simulink model "Demo_DSRC_BSM_I_and_II_Message_cs"  (Simulink 7.6)
settings: Solver=ode5  SolverMode=SingleTasking  StartTime=0.0  StopTime=40  FixedStep=1/20  RelTol=1e-3
PreLoadFcn:
  | check_NUTS_defined;
  | 
  | assignin('base',['model_closed_' bdroot],false);
InitFcn:
  | PreScanExperimentInitFcn(bdroot)
StopFcn:
  | PreScanExperimentStopFcn(bdroot)
libraries: simulink x9, PreScanSimulinkLibrary x8, PreScanUsefulBlocks x5, simulink_extras x1
(part 2 of 3)

== system Demo_DSRC_BSM_I_and_II_Message_cs/Mazda_RX8_1/Basic Safety Message II ==
  ThrottlePosition : Inport
  ExteriorLights : Inport  Port=2
  CrumbData : Inport  Port=3
  itemCnt : Inport  Port=4
  Confidence : Inport  Port=5
  RadiusOfCurve : Inport  Port=6
  EventFlag : Inport  Port=7
  BSM-II Creator : Subsystem  InitFcn=|  StopFcn=|
      InitFcn=|
      | clear elems;
      | elems(1) = Simulink.BusElement;
      | elems(1).Name = 'VehicleStatus';
      | elems(1).Dimensions = 1;
      | elems(1).DataType = 'VehicleStatus';
      | elems(1).SampleTime = -1;
      | elems(1).Complexity = 'real';
      | elems(1).SamplingMode = 'Sample based';
      | elems(2) = Simulink.BusElement;
      | elems(2).Name = 'VehicleSafetyExtension';
      | elems(2).Dimensions = 1;
      | elems(2).DataType = 'VehicleSafetyExtension';
      | elems(2).SampleTime = -1;
      | elems(2).Complexity = 'real';
      | elems(2).SamplingMode = 'Sample based';
      | BSMII = Simulink.Bus;
      | BSMII.HeaderFile = '';
      | BSMII.Description = sprintf('BSMII message set');
      | BSMII.Elements = elems;
      | assignin('base', 'BSMII', BSMII)
      | % Bus object: PathHistory
      | clear elems;
      | elems(1) = Simulink.BusElement;
      | elems(1).Name = 'CrumbData';
      | elems(1).Dimensions = 184;
      | elems(1).DataType = 'uint8';
      | elems(1).SampleTime = -1;
      | elems(1).Complexity = 'real';
      | elems(1).SamplingMode = 'Sample based';
      | elems(2) = Simulink.BusElement;
      | elems(2).Name = 'itemCnt';
      | elems(2).Dimensions = 1;
      | elems(2).DataType = 'uint8';
      | elems(2).SampleTime = -1;
      | elems(2).Complexity = 'real';
      | elems(2).SamplingMode = 'Sample based';
      | PathHistory = Simulink.Bus;
      | PathHistory.HeaderFile = '';
      | PathHistory.Description = sprintf('');
      | PathHistory.Elements = elems;
      | assignin('base', 'PathHistory', PathHistory)
      | % Bus object: PathPrediction
      | clear elems;
      | elems(1) = Simulink.BusElement;
      | elems(1).Name = 'Confidence';
      | elems(1).Dimensions = 1;
      | elems(1).DataType = 'uint8';
      | elems(1).SampleTime = -1;
      | elems(1).Complexity = 'real';
      | elems(1).SamplingMode = 'Sample based';
      | elems(2) = Simulink.BusElement;
      | elems(2).Name = 'RadiusOfCurve';
      | elems(2).Dimensions = 1;
      | elems(2).DataType = 'int16';
      | elems(2).SampleTime = -1;
      | elems(2).Complexity = 'real';
      | elems(2).SamplingMode = 'Sample based';
      | PathPrediction = Simulink.Bus;
      | PathPrediction.HeaderFile = '';
      | PathPrediction.Description = sprintf('');
      | PathPrediction.Elements = elems;
      | assignin('base', 'PathPrediction', PathPrediction)
      | % Bus object: VehicleSafetyExtension
      | clear elems;
      | elems(1) = Simulink.BusElement;
      | elems(1).Name = 'PathPrediction';
      | elems(1).Dimensions = 1;
      | elems(1).DataType = 'PathPrediction';
      | elems(1).SampleTime = -1;
      | elems(1).Complexity = 'real';
      | elems(1).SamplingMode = 'Sample based';
      | elems(2) = Simulink.BusElement;
      | elems(2).Name = 'PathHistory';
      | elems(2).Dimensions = 1;
      | elems(2).DataType = 'PathHistory';
      | elems(2).SampleTime = -1;
      | elems(2).Complexity = 'real';
      | elems(2).SamplingMode = 'Sample based';
      | elems(3) = Simulink.BusElement;
      | elems(3).Name = 'EventFlag';
      | elems(3).Dimensions = 1;
      | elems(3).DataType = 'uint32';
      | elems(3).SampleTime = -1;
      | elems(3).Complexity = 'real';
      | elems(3).SamplingMode = 'Sample based';
      | VehicleSafetyExtension = Simulink.Bus;
      | VehicleSafetyExtension.HeaderFile = '';
      | VehicleSafetyExtension.Description = sprintf('');
      | VehicleSafetyExtension.Elements = elems;
      | assignin('base', 'VehicleSafetyExtension', VehicleSafetyExtension)
      | % Bus object: VehicleStatus
      | clear elems;
      | elems(1) = Simulink.BusElement;
      | elems(1).Name = 'ThrottlePosition';
      | elems(1).Dimensions = 1;
      | elems(1).DataType = 'uint8';
      | elems(1).SampleTime = -1;
      | elems(1).Complexity = 'real';
      | elems(1).SamplingMode = 'Sample based';
      | elems(2) = Simulink.BusElement;
      | elems(2).Name = 'ExteriorLights';
      | elems(2).Dimensions = 1;
      | elems(2).DataType = 'uint8';
      | elems(2).SampleTime = -1;
      | elems(2).Complexity = 'real';
      | elems(2).SamplingMode = 'Sample based';
      | VehicleStatus = Simulink.Bus;
      | VehicleStatus.HeaderFile = '';
      | VehicleStatus.Description = sprintf('');
      | VehicleStatus.Elements = elems;
      | assignin('base', 'VehicleStatus', VehicleStatus)
      StopFcn=|
      | clear BSMII
      | clear PathHistory
      | clear PathPrediction
      | clear VehicleSafetyExtension
      | clear VehicleStatus
      | clear elems
  BSM-II Unpacker : Subsystem
  Bus Creator : BusCreator  Inputs=8
  Enabled Basic Safety Message I and II : Subsystem
  BSMII : Outport
  wires:
  Enabled Basic Safety Message I and II/8(CrumbData out) -> Bus Creator/8  "CrumbData"
  Enabled Basic Safety Message I and II/7(Throttle position out) -> Bus Creator/7  "ThrottlePosition"
  Enabled Basic Safety Message I and II/6(Exterior lights out) -> Bus Creator/6  "ExteriorLights"
  Enabled Basic Safety Message I and II/5(Confidence out) -> Bus Creator/5  "Confidence"
  Enabled Basic Safety Message I and II/4(radius of Curve out) -> Bus Creator/4  "RadiusOfCurve"
  Enabled Basic Safety Message I and II/3(item Count out) -> Bus Creator/3  "itemCnt"
  Enabled Basic Safety Message I and II/2(Eventflag out) -> Bus Creator/2  "EventFlag"
  Enabled Basic Safety Message I and II/1(Enabled descriptor out) -> Bus Creator/1  "Enabled descriptor"
  BSM-II Creator/1(BSMII) -> BSM-II Unpacker/1(BSMII)
  Bus Creator/1 -> BSMII/1  "BSMII"
  ThrottlePosition/1 -> BSM-II Creator/1(ThrottlePositon)  "ThrottlePosition"
  ExteriorLights/1 -> BSM-II Creator/2(ExteriorLights)  "ExteriorLights"
  CrumbData/1 -> BSM-II Creator/3(CrumbData)  "CrumbData"
  itemCnt/1 -> BSM-II Creator/4(itemCnt)  "itemCnt"
  Confidence/1 -> BSM-II Creator/5(Confidence)  "Confidence"
  RadiusOfCurve/1 -> BSM-II Creator/6(RadiusOfCurve)  "RadiusOfCurve"
  EventFlag/1 -> BSM-II Creator/7(EventFlag)  "EventFlag"
  BSM-II Unpacker/1(Eventflag) -> Enabled Basic Safety Message I and II/1(Eventflag in)
  BSM-II Unpacker/2(itemCnt) -> Enabled Basic Safety Message I and II/2(itemCnt in)
  BSM-II Unpacker/3(RadiusOfCurve) -> Enabled Basic Safety Message I and II/3(radiusOfCurve in)
  BSM-II Unpacker/4(Confidence) -> Enabled Basic Safety Message I and II/4(Confidence in)
  BSM-II Unpacker/5(ExteriorLights) -> Enabled Basic Safety Message I and II/5(Exterior lights in)
  BSM-II Unpacker/6(ThrottlePosition) -> Enabled Basic Safety Message I and II/6(Throttle position in)
  BSM-II Unpacker/7(CrumbData_DoubleVector) -> Enabled Basic Safety Message I and II/7(CrumbData in)

== system Demo_DSRC_BSM_I_and_II_Message_cs/Mazda_RX8_1/DSRC Transmitter BSM I and II ==
  Data1 : Inport
  Enable : EnablePort  PropagateVarSize=During execution
  Always Enabled1 : Constant
  DSRC_T_BusAssignment : BusAssignment  Tag=BusDSRCT  AssignedSignals=spare_1,spare_2,spare_3,spare_4,spare_5,spare_6,spare_7,spare_8,spare_9,spare_10,spare_11,spare_12,spare_13,spare_14,spare_15,spare_16,spare_17,spare_18,spare_19,spare_20,spare_21,spare_22,spare_23,spare_24,spare_25,spare_26,spare_27,spare_28,spare_29,spare_30,spare_31,spare_32,spare_33,spare_34,spare_35,spare_36,spare_37,spare_38,spare_39,spare_40,spare_41,spare_42,spare_43,spare_44,spare_45,spare_46,spare_47,spare_48,spare_49,spare_50,spare_51,spare_52,spare_53,spare_54,spare_55,spare_56,spare_57,spare_58,spare_59,spare_60,spare_61,spare_62,spare_63
  DSRC_T_Mux : Subsystem  Tag=MuxDSRCT
      settings: DeleteFcn=PreScanBlockDeleteFcn;
      mask Type: PreScan Mux Block:
      mask Display:
      | port_label('input', 1, 'Warning signal ID')
      | port_label('input', 2, 'Maneuvre ID')
      | port_label('input', 3, 'Vehicle Type')
      | port_label('input', 4, 'Braking Capacity')
      | port_label('input', 5, 'Vehicle Size')
      | port_label('input', 6, 'spare')
  Demux : Demux  Outputs=63
  Ground_{4..8} (5 alike) : Ground
  DSRC_T : Outport  Tag=AntennaTOutport
  f() : Outport  Port=2  InitialOutput=[1]
  wires:
  DSRC_T_Mux/2(Out2) -> DSRC_T_BusAssignment/1  "L29"
  DSRC_T_Mux/1(Out1) -> DSRC_T/1  "l60"
  Ground_4/1 -> DSRC_T_Mux/1(warning_signal_id)  "l46"
  Ground_5/1 -> DSRC_T_Mux/2(maneuvre_id)  "l47"
  Ground_6/1 -> DSRC_T_Mux/3(vehicle_type)  "l48"
  Ground_7/1 -> DSRC_T_Mux/4(brakingcapacity)  "l49"
  Ground_8/1 -> DSRC_T_Mux/5(vehicle_size)  "l50"
  Demux/39 -> DSRC_T_BusAssignment/40
  Always Enabled1/1 -> f()/1
  DSRC_T_BusAssignment/1 -> DSRC_T_Mux/6(spare)  "l58"
  Demux/1 -> DSRC_T_BusAssignment/2  "MsgId"
  Demux/2 -> DSRC_T_BusAssignment/3  "MsgCount"
  Demux/3 -> DSRC_T_BusAssignment/4  "TempId"
  Demux/4 -> DSRC_T_BusAssignment/5  "SecMark"
  Demux/5 -> DSRC_T_BusAssignment/6  "Lateral"
  Demux/6 -> DSRC_T_BusAssignment/7  "Longitudinal"
  Demux/7 -> DSRC_T_BusAssignment/8  "Elevation"
  Demux/8 -> DSRC_T_BusAssignment/9  "Accuracy"
  Demux/9 -> DSRC_T_BusAssignment/10  "Transmission State"
  Demux/10 -> DSRC_T_BusAssignment/11  "Speed"
  Demux/11 -> DSRC_T_BusAssignment/12  "Heading"
  Demux/12 -> DSRC_T_BusAssignment/13  "Angle"
  Demux/13 -> DSRC_T_BusAssignment/14  "Longitudinal Acc"
  Demux/14 -> DSRC_T_BusAssignment/15  "Lateral Acc"
  Demux/15 -> DSRC_T_BusAssignment/16  "Veritical Acc"
  Demux/16 -> DSRC_T_BusAssignment/17  "Yaw rate"
  Demux/17 -> DSRC_T_BusAssignment/18  "Brakes"
  Demux/18 -> DSRC_T_BusAssignment/19  "Vehicle Width"
  Demux/19 -> DSRC_T_BusAssignment/20  "Vehicle Height"
  Demux/20 -> DSRC_T_BusAssignment/21  "Enabled_Descriptor"
  Demux/21 -> DSRC_T_BusAssignment/22  "Eventflag"
  Demux/22 -> DSRC_T_BusAssignment/23  "itemCnt"
  Demux/23 -> DSRC_T_BusAssignment/24  "radiusOfCurve"
  Demux/24 -> DSRC_T_BusAssignment/25  "confidence"
  Demux/25 -> DSRC_T_BusAssignment/26  "Exterior lights"
  Demux/26 -> DSRC_T_BusAssignment/27  "Throttle position"
  Demux/27 -> DSRC_T_BusAssignment/28
  Demux/28 -> DSRC_T_BusAssignment/29
  Demux/29 -> DSRC_T_BusAssignment/30
  Data1/1 -> Demux/1
  Demux/30 -> DSRC_T_BusAssignment/31
  Demux/31 -> DSRC_T_BusAssignment/32
  Demux/32 -> DSRC_T_BusAssignment/33
  Demux/33 -> DSRC_T_BusAssignment/34
  Demux/34 -> DSRC_T_BusAssignment/35
  Demux/35 -> DSRC_T_BusAssignment/36
  Demux/36 -> DSRC_T_BusAssignment/37
  Demux/37 -> DSRC_T_BusAssignment/38
  Demux/38 -> DSRC_T_BusAssignment/39
  Demux/40 -> DSRC_T_BusAssignment/41
  Demux/41 -> DSRC_T_BusAssignment/42
  Demux/42 -> DSRC_T_BusAssignment/43
  Demux/43 -> DSRC_T_BusAssignment/44
  Demux/44 -> DSRC_T_BusAssignment/45
  Demux/45 -> DSRC_T_BusAssignment/46
  Demux/46 -> DSRC_T_BusAssignment/47
  Demux/47 -> DSRC_T_BusAssignment/48
  Demux/48 -> DSRC_T_BusAssignment/49
  Demux/49 -> DSRC_T_BusAssignment/50
  Demux/50 -> DSRC_T_BusAssignment/51
  Demux/51 -> DSRC_T_BusAssignment/52
  Demux/52 -> DSRC_T_BusAssignment/53
  Demux/53 -> DSRC_T_BusAssignment/54
  Demux/54 -> DSRC_T_BusAssignment/55
  Demux/55 -> DSRC_T_BusAssignment/56
  Demux/56 -> DSRC_T_BusAssignment/57
  Demux/57 -> DSRC_T_BusAssignment/58
  Demux/58 -> DSRC_T_BusAssignment/59
  Demux/59 -> DSRC_T_BusAssignment/60
  Demux/60 -> DSRC_T_BusAssignment/61
  Demux/61 -> DSRC_T_BusAssignment/62
  Demux/62 -> DSRC_T_BusAssignment/63
  Demux/63 -> DSRC_T_BusAssignment/64

== system Demo_DSRC_BSM_I_and_II_Message_cs/Mazda_RX8_1/J2735 Encoder Basic Safety Message I and II ==
  Msg : Inport
  Enable : EnablePort  PropagateVarSize=During execution
  Always Enabled : Constant
  Bus Selector : BusSelector  OutputSignals=Enabled descriptor,EventFlag,itemCnt,RadiusOfCurve,Confidence,ExteriorLights,ThrottlePosition,CrumbData
  Bus Selector1 : BusSelector  OutputSignals=BSMI,BSMII
  Demux : Demux  Outputs=19
  Demux2 : Demux  Outputs=37
  Embedded MATLAB Function : Stateflow chart  TreatAsAtomicUnit=on
  f() : Outport  InitialOutput=[1]
  Data : Outport  Port=2
  wires:
  Always Enabled/1 -> f()/1
  Embedded MATLAB Function/1(y) -> Data/1
  Demux/19 -> Embedded MATLAB Function/19(u19)
  Demux/18 -> Embedded MATLAB Function/18(u18)
  Demux/17 -> Embedded MATLAB Function/17(u17)
  Demux/16 -> Embedded MATLAB Function/16(u16)
  Demux/15 -> Embedded MATLAB Function/15(u15)
  Demux/14 -> Embedded MATLAB Function/14(u14)
  Demux/13 -> Embedded MATLAB Function/13(u13)
  Demux/12 -> Embedded MATLAB Function/12(u12)
  Demux/11 -> Embedded MATLAB Function/11(u11)
  Demux/10 -> Embedded MATLAB Function/10(u10)
  Demux/9 -> Embedded MATLAB Function/9(u9)
  Demux/8 -> Embedded MATLAB Function/8(u8)
  Demux/7 -> Embedded MATLAB Function/7(u7)
  Demux/6 -> Embedded MATLAB Function/6(u6)
  Demux/5 -> Embedded MATLAB Function/5(u5)
  Demux/4 -> Embedded MATLAB Function/4(u4)
  Demux/3 -> Embedded MATLAB Function/3(u3)
  Demux/2 -> Embedded MATLAB Function/2(u2)
  Demux/1 -> Embedded MATLAB Function/1(u1)
  Bus Selector/3 -> Embedded MATLAB Function/22(u22)  "<itemCnt>"
  Bus Selector/4 -> Embedded MATLAB Function/23(u23)  "<RadiusOfCurve>"
  Bus Selector/5 -> Embedded MATLAB Function/24(u24)  "<Confidence>"
  Bus Selector/6 -> Embedded MATLAB Function/25(u25)  "<ExteriorLights>"
  Bus Selector/7 -> Embedded MATLAB Function/26(u26)  "<ThrottlePosition>"
  Demux2/1 -> Embedded MATLAB Function/27(u27)  "CrumbData1"
  Demux2/2 -> Embedded MATLAB Function/28(u28)  "CrumbData2"
  Demux2/3 -> Embedded MATLAB Function/29(u29)  "CrumbData3"
  Bus Selector/8 -> Demux2/1  "<CrumbData>"
  Demux2/4 -> Embedded MATLAB Function/30(u30)  "CrumbData4"
  Demux2/5 -> Embedded MATLAB Function/31(u31)  "CrumbData5"
  Demux2/6 -> Embedded MATLAB Function/32(u32)  "CrumbData6"
  Demux2/7 -> Embedded MATLAB Function/33(u33)  "CrumbData7"
  Demux2/8 -> Embedded MATLAB Function/34(u34)  "CrumbData8"
  Demux2/9 -> Embedded MATLAB Function/35(u35)  "CrumbData9"
  Demux2/10 -> Embedded MATLAB Function/36(u36)  "crumbData10"
  Demux2/11 -> Embedded MATLAB Function/37(u37)  "CrumbData11"
  Demux2/12 -> Embedded MATLAB Function/38(u38)  "CrumbData12"
  Demux2/13 -> Embedded MATLAB Function/39(u39)  "CrumbData13"
  Demux2/14 -> Embedded MATLAB Function/40(u40)  "CrumbData14"
  Demux2/15 -> Embedded MATLAB Function/41(u41)  "CrumbData15"
  Demux2/16 -> Embedded MATLAB Function/42(u42)  "CrumbData16"
  Demux2/17 -> Embedded MATLAB Function/43(u43)  "CrumbData17"
  Demux2/18 -> Embedded MATLAB Function/44(u44)  "CrumbData18"
  Demux2/19 -> Embedded MATLAB Function/45(u45)  "CrumbData19"
  Demux2/20 -> Embedded MATLAB Function/46(u46)  "CrumbData20"
  Demux2/21 -> Embedded MATLAB Function/47(u47)  "CrumbData21"
  Demux2/22 -> Embedded MATLAB Function/48(u48)  "CrumbData22"
  Demux2/23 -> Embedded MATLAB Function/49(u49)  "CrumbData23"
  Demux2/24 -> Embedded MATLAB Function/50(u50)  "CrumbData24"
  Demux2/25 -> Embedded MATLAB Function/51(u51)  "CrumbData25"
  Demux2/26 -> Embedded MATLAB Function/52(u52)  "CrumbData26"
  Demux2/27 -> Embedded MATLAB Function/53(u53)  "CrumbData27"
  Demux2/28 -> Embedded MATLAB Function/54(u54)  "CrumbData28"
  Demux2/29 -> Embedded MATLAB Function/55(u55)  "CrumbData29"
  Demux2/30 -> Embedded MATLAB Function/56(u56)  "CrumbData30"
  Demux2/31 -> Embedded MATLAB Function/57(u57)  "CrumbData31"
  Demux2/32 -> Embedded MATLAB Function/58(u58)  "CrumbData32"
  Demux2/33 -> Embedded MATLAB Function/59(u59)  "CrumbData33"
  Demux2/34 -> Embedded MATLAB Function/60(u60)  "CrumbData34"
  Demux2/35 -> Embedded MATLAB Function/61(u61)  "CrumbData35"
  Demux2/36 -> Embedded MATLAB Function/62(u62)  "CrumbData36"
  Demux2/37 -> Embedded MATLAB Function/63(u63)  "CrumbData37"
  Msg/1 -> Bus Selector1/1
  Bus Selector1/1 -> Demux/1  "<BSMI>"
  Bus Selector1/2 -> Bus Selector/1  "<BSMII>"
  Bus Selector/1 -> Embedded MATLAB Function/20(u20)  "<Enabled descriptor>"
  Bus Selector/2 -> Embedded MATLAB Function/21(u21)  "<EventFlag>"

== system Demo_DSRC_BSM_I_and_II_Message_cs/Mazda_RX8_1/Radius and confidence computation ==
  Lat1 [deg] : Inport
  Long1 [deg] : Inport  Port=2
  Altitude1 [m] : Inport  Port=3
  Heading1 [deg] : Inport  Port=4
  Yaw rate [deg/s] : Inport  Port=5
  Center point of the bend : Subsystem
  Confidence level : Subsystem
  Degrees2Radians : Subsystem
  GPS2xyz1 : PreScanUsefulBlocks/GPS2xyz  CoordinateCount=1  GPS_base=GPS_origin
  GPS2xyz2 : PreScanUsefulBlocks/GPS2xyz  CoordinateCount=1  GPS_base=GPS_origin
  Heading angle conversion : Subsystem
  Limitations : Subsystem
  Mux : Mux  Inputs=3
  Mux1 : Mux  Inputs=3
  Previous reading : Subsystem
  Radius computation : Subsystem
  Rate transition : Subsystem
  Selector : Selector  InputPortWidth=3  IndexOptions=Index vector (dialog)  Indices=[1 2]  OutputSizes=1
  Selector1 : Selector  InputPortWidth=3  IndexOptions=Index vector (dialog)  Indices=[1 2]  OutputSizes=1
  Radius [m] : Outport
  Center [xp,yp] : Outport  Port=2
  Confidence [%] : Outport  Port=3
  wires:
  Radius computation/2(delta_Phi) -> Center point of the bend/2(delta_Phi), Limitations/2(d_Phi)
  Mux1/1 -> GPS2xyz2/1
  Mux/1 -> GPS2xyz1/1
  Degrees2Radians/6(heading2r) -> Radius computation/6(heading2)
  Degrees2Radians/5(long2r) -> Radius computation/5(long2)
  Degrees2Radians/4(lat2r) -> Radius computation/4(lat2)
  Degrees2Radians/3(heading1r) -> Radius computation/3(heading1)
  Degrees2Radians/2(long1r) -> Radius computation/2(Iong1)
  Degrees2Radians/1(lat1r) -> Radius computation/1(Iat1)
  GPS2xyz1/1 -> Selector/1
  GPS2xyz2/1 -> Selector1/1
  Selector/1 -> Center point of the bend/3("[x1,y1]")
  Selector1/1 -> Center point of the bend/4("[x2,y2]")
  Lat1 [deg]/1 -> Rate transition/1(Lat_in [deg])
  Long1 [deg]/1 -> Rate transition/2(Long_in [deg])
  Altitude1 [m]/1 -> Rate transition/3(Alt_in [m])
  Heading1 [deg]/1 -> Rate transition/4(Heading_in [deg])
  Rate transition/3(Heading [deg]) -> Heading angle conversion/1(H_in [deg])
  Rate transition/1(Lat [deg]) -> Previous reading/1(Lat_in [deg]), Degrees2Radians/1(Iat1d), Mux/1
  Rate transition/2(Long [deg]) -> Previous reading/2(Long_in [deg]), Degrees2Radians/2(Iong1d), Mux/2
  Heading angle conversion/1(H_out [deg]) -> Degrees2Radians/3(heading1d), Previous reading/3(Heading_in [deg])
  Rate transition/4(Alt [m]) -> Previous reading/4(Alt_in [m]), Mux/3
  Previous reading/1(Lat2 [deg]) -> Degrees2Radians/4(lat2d), Mux1/1
  Previous reading/2(Long2 [deg]) -> Degrees2Radians/5(long2d), Mux1/2
  Previous reading/3(Heading2 [deg]) -> Degrees2Radians/6(heading2d)
  Previous reading/4(Alt2 [m]) -> Mux1/3
  Radius computation/1(Radius) -> Center point of the bend/1(R), Limitations/1(R)
  Center point of the bend/1(Center point) -> Limitations/3("[xp,yp]")
  Limitations/1(Radius [m]) -> Radius [m]/1
  Limitations/2(Center point) -> Center [xp,yp]/1
  Yaw rate [deg/s]/1 -> Confidence level/1(Yaw rate [deg/s])
  Confidence level/1(Confidence [%]) -> Confidence [%]/1

== system Demo_DSRC_BSM_I_and_II_Message_cs/Mazda_RX8_1/SELF_Demux ==
  SELF : Inport
  Demux1 : Demux  Outputs=3
  Demux2 : Demux  Outputs=3
  Demux3 : Demux  Outputs=[3 3 1 1]
  Demux4 : Demux  Outputs=3
  Gain : Gain  Gain=180/pi
  Gain1 : Gain  Gain=180/pi
  Selector : Selector  InputPortWidth=3  IndexOptions=Index vector (dialog)  Indices=[3]  OutputSizes=1
  compas converter : Subsystem
  xyz2GPS : PreScanUsefulBlocks/xyz2GPS  CoordinateCount=1  GPS_base=[0.000000 0.000000 0.000]
  x [m] : Outport
  y [m] : Outport  Port=2
  z [m] : Outport  Port=3
  rotx [deg] : Outport  Port=4
  roty [deg] : Outport  Port=5
  rotz [deg] : Outport  Port=6
  GPS lat [deg] : Outport  Port=7
  GPS long [deg] : Outport  Port=8
  GPS alt [m] : Outport  Port=9
  velocity [m/s] : Outport  Port=10
  heading [deg] : Outport  Port=11
  yaw rate [deg/s] : Outport  Port=12
  wires:
  Demux3/4 -> Gain1/1
  Gain1/1 -> yaw rate [deg/s]/1
  Demux3/3 -> velocity [m/s]/1
  compas converter/1(heading [deg]) -> heading [deg]/1
  xyz2GPS/1 -> Demux4/1
  Demux4/3 -> GPS alt [m]/1
  Demux4/2 -> GPS long [deg]/1
  Demux4/1 -> GPS lat [deg]/1
  Demux3/2 -> Gain/1, Selector/1
  Demux3/1 -> xyz2GPS/1, Demux1/1
  SELF/1 -> Demux3/1
  Demux2/3 -> rotz [deg]/1
  Demux2/2 -> roty [deg]/1
  Demux2/1 -> rotx [deg]/1
  Demux1/3 -> z [m]/1
  Demux1/2 -> y [m]/1
  Demux1/1 -> x [m]/1
  Gain/1 -> Demux2/1
  Selector/1 -> compas converter/1(rotz [rad])

== system Demo_DSRC_BSM_I_and_II_Message_cs/Mazda_RX8_1/Trajectories ==
  Traj2State1 : Subsystem  Tag=Traj2State
      settings: DeleteFcn=PreScanBlockDeleteFcn;
      mask Type: PreScan Demux Block:
  Trajectory_1 : Subsystem  Tag=Trajectory  mask(PreScan Source Block: Trajectory){FileName='Trajectory_1.mat', TimeStep=1/20}
      mask prompts: TimeStep "Time Step [s]"
      mask help:
      | The Trajectory block contains the trajectories defined in the PreScan Experiment Editor. The output of the trajectory block is the (vehicle) State.
      |
      | For more information, please click Help.
      mask init: same as Demo_DSRC_BSM_I_and_II_Message_cs/Ford_Fiesta_1/Trajectories/Trajectory_2
      settings: DeleteFcn=PreScanBlockDeleteFcn;
      mask Help: eval('openHelp(312)')
      mask Display: fprintf(FileName)
  Trajectory_1_Offset : Constant  Tag=TrajectoryOffset  Value="[0  0  0  0  0  0]"
  State : Outport  Tag=TrajOutport
  wires:
  Trajectory_1/1(trajectory) -> Traj2State1/1(Traj Org)
  Trajectory_1_Offset/1 -> Traj2State1/2(Offset)
  Traj2State1/1(state) -> State/1

== system Demo_DSRC_BSM_I_and_II_Message_cs/STATE_Ford_Fiesta_1/Acceleration ==
  Y : Inport
  Assignment : Assignment  IndexMode=Zero-based  SampleTime=TimeStep  IndexOptions=Starting index (dialog)  Indices=PortIndex  OutputSizes=[1 1]
  Data Store Read : DataStoreRead  DataStoreName=SimCoreActuators  SampleTime=TimeStep
  Data Store Write : DataStoreWrite  DataStoreName=SimCoreActuators
  wires:
  Assignment/1 -> Data Store Write/1
  Data Store Read/1 -> Assignment/1
  Y/1 -> Assignment/2

== system Demo_DSRC_BSM_I_and_II_Message_cs/STATE_Ford_Fiesta_1/Position ==
  Y : Inport
  Assignment : Assignment  IndexMode=Zero-based  SampleTime=TimeStep  IndexOptions=Starting index (dialog)  Indices=PortIndex  OutputSizes=[1 1]
  Data Store Read : DataStoreRead  DataStoreName=SimCoreActuators  SampleTime=TimeStep
  Data Store Write : DataStoreWrite  DataStoreName=SimCoreActuators
  wires:
  Y/1 -> Assignment/2
  Data Store Read/1 -> Assignment/1
  Assignment/1 -> Data Store Write/1

== system Demo_DSRC_BSM_I_and_II_Message_cs/STATE_Ford_Fiesta_1/RPY ==
  Y : Inport
  Assignment : Assignment  IndexMode=Zero-based  SampleTime=TimeStep  IndexOptions=Starting index (dialog)  Indices=PortIndex  OutputSizes=[1 1]
  Data Store Read : DataStoreRead  DataStoreName=SimCoreActuators  SampleTime=TimeStep
  Data Store Write : DataStoreWrite  DataStoreName=SimCoreActuators
  wires:
  Assignment/1 -> Data Store Write/1
  Data Store Read/1 -> Assignment/1
  Y/1 -> Assignment/2

== system Demo_DSRC_BSM_I_and_II_Message_cs/STATE_Ford_Fiesta_1/Velocity ==
  Y : Inport
  Assignment : Assignment  IndexMode=Zero-based  SampleTime=TimeStep  IndexOptions=Starting index (dialog)  Indices=PortIndex  OutputSizes=[1 1]
  Data Store Read : DataStoreRead  DataStoreName=SimCoreActuators  SampleTime=TimeStep
  Data Store Write : DataStoreWrite  DataStoreName=SimCoreActuators
  wires:
  Assignment/1 -> Data Store Write/1
  Data Store Read/1 -> Assignment/1
  Y/1 -> Assignment/2

== system Demo_DSRC_BSM_I_and_II_Message_cs/STATE_Ford_Fiesta_1/velRPY ==
  Y : Inport
  Assignment : Assignment  IndexMode=Zero-based  SampleTime=TimeStep  IndexOptions=Starting index (dialog)  Indices=PortIndex  OutputSizes=[1 1]
  Data Store Read : DataStoreRead  DataStoreName=SimCoreActuators  SampleTime=TimeStep
  Data Store Write : DataStoreWrite  DataStoreName=SimCoreActuators
  wires:
  Assignment/1 -> Data Store Write/1
  Data Store Read/1 -> Assignment/1
  Y/1 -> Assignment/2

== system Demo_DSRC_BSM_I_and_II_Message_cs/STATE_Mazda_RX8_1/Acceleration ==
  Y : Inport
  Assignment : Assignment  IndexMode=Zero-based  SampleTime=TimeStep  IndexOptions=Starting index (dialog)  Indices=PortIndex  OutputSizes=[1 1]
  Data Store Read : DataStoreRead  DataStoreName=SimCoreActuators  SampleTime=TimeStep
  Data Store Write : DataStoreWrite  DataStoreName=SimCoreActuators
  wires:
  Assignment/1 -> Data Store Write/1
  Data Store Read/1 -> Assignment/1
  Y/1 -> Assignment/2

== system Demo_DSRC_BSM_I_and_II_Message_cs/STATE_Mazda_RX8_1/Position ==
  Y : Inport
  Assignment : Assignment  IndexMode=Zero-based  SampleTime=TimeStep  IndexOptions=Starting index (dialog)  Indices=PortIndex  OutputSizes=[1 1]
  Data Store Read : DataStoreRead  DataStoreName=SimCoreActuators  SampleTime=TimeStep
  Data Store Write : DataStoreWrite  DataStoreName=SimCoreActuators
  wires:
  Y/1 -> Assignment/2
  Data Store Read/1 -> Assignment/1
  Assignment/1 -> Data Store Write/1

== system Demo_DSRC_BSM_I_and_II_Message_cs/STATE_Mazda_RX8_1/RPY ==
  Y : Inport
  Assignment : Assignment  IndexMode=Zero-based  SampleTime=TimeStep  IndexOptions=Starting index (dialog)  Indices=PortIndex  OutputSizes=[1 1]
  Data Store Read : DataStoreRead  DataStoreName=SimCoreActuators  SampleTime=TimeStep
  Data Store Write : DataStoreWrite  DataStoreName=SimCoreActuators
  wires:
  Assignment/1 -> Data Store Write/1
  Data Store Read/1 -> Assignment/1
  Y/1 -> Assignment/2

== system Demo_DSRC_BSM_I_and_II_Message_cs/STATE_Mazda_RX8_1/Velocity ==
  Y : Inport
  Assignment : Assignment  IndexMode=Zero-based  SampleTime=TimeStep  IndexOptions=Starting index (dialog)  Indices=PortIndex  OutputSizes=[1 1]
  Data Store Read : DataStoreRead  DataStoreName=SimCoreActuators  SampleTime=TimeStep
  Data Store Write : DataStoreWrite  DataStoreName=SimCoreActuators
  wires:
  Assignment/1 -> Data Store Write/1
  Data Store Read/1 -> Assignment/1
  Y/1 -> Assignment/2

== system Demo_DSRC_BSM_I_and_II_Message_cs/STATE_Mazda_RX8_1/velRPY ==
  Y : Inport
  Assignment : Assignment  IndexMode=Zero-based  SampleTime=TimeStep  IndexOptions=Starting index (dialog)  Indices=PortIndex  OutputSizes=[1 1]
  Data Store Read : DataStoreRead  DataStoreName=SimCoreActuators  SampleTime=TimeStep
  Data Store Write : DataStoreWrite  DataStoreName=SimCoreActuators
  wires:
  Assignment/1 -> Data Store Write/1
  Data Store Read/1 -> Assignment/1
  Y/1 -> Assignment/2

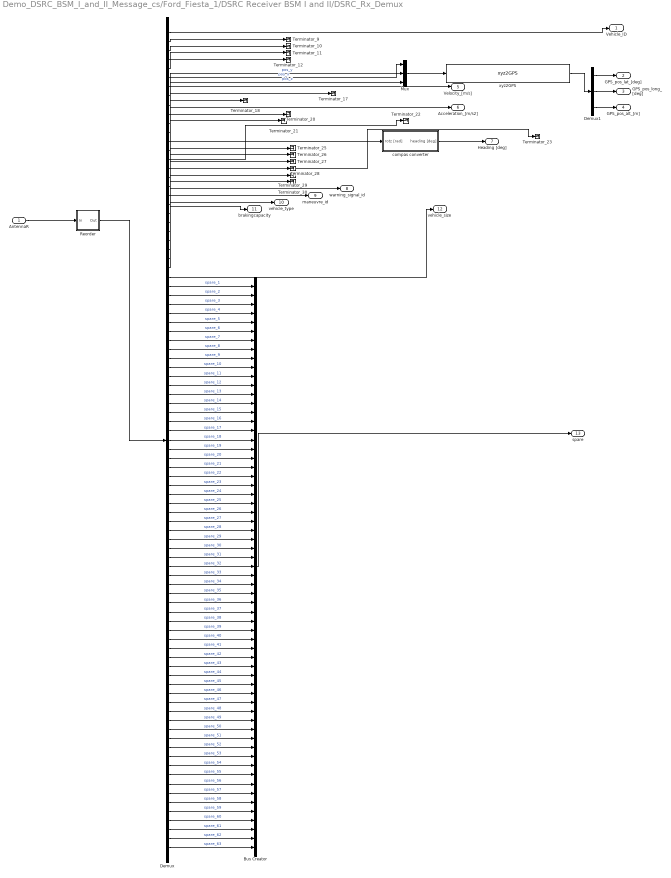
== system Demo_DSRC_BSM_I_and_II_Message_cs/Ford_Fiesta_1/DSRC Receiver BSM I and II/DSRC_Rx_Demux ==
  AntennaR : Inport
  Bus Creator : BusCreator  Inputs=63
  Demux : Demux  Outputs=91
  Demux1 : Demux  Outputs=3
  Mux : Mux  Inputs=3
  Reorder : Subsystem  mask(Output reorder block){NrOfOutputs=91, NrOfObjects=1}
      mask prompts: NrOfOutputs "Number Of Outputs [-]"; NrOfObjects "Number Of Objects [-]"
      mask help: Change output order from object based to output type based
      mask init:
      | InputPortWidth=NrOfObjects*NrOfOutputs;
      | Input=1:InputPortWidth;
      | ReshapedInput=reshape(Input,NrOfOutputs,NrOfObjects);
      | TransposedReshapedInput=transpose(ReshapedInput);
      | Elements=reshape(TransposedReshapedInput,length(Input),1);
  Terminator_{9..12,17..18,20..23,25..30} (16 alike) : Terminator
  compas converter : Subsystem
  xyz2GPS : PreScanUsefulBlocks/xyz2GPS  CoordinateCount=1  GPS_base=[0.000000 0.000000 0.000]
  Vehicle_ID : Outport
  GPS_pos_lat_[deg] : Outport  Port=2
  GPS_pos_long_[deg] : Outport  Port=3
  GPS_pos_alt_[m] : Outport  Port=4
  Velocity_[m/s] : Outport  Port=5
  Acceleration_[m/s2] : Outport  Port=6
  Heading [deg] : Outport  Port=7
  warning_signal_id : Outport  Port=8
  maneuvre_id : Outport  Port=9
  vehicle_type : Outport  Port=10
  brakingcapacity : Outport  Port=11
  vehicle_size : Outport  Port=12
  spare : Outport  Port=13
  wires:
  Bus Creator/1 -> spare/1
  compas converter/1(heading [deg]) -> Heading [deg]/1
  Demux/1 -> Vehicle_ID/1
  Demux/2 -> Terminator_9/1
  Demux/3 -> Terminator_10/1
  Demux/4 -> Terminator_11/1
  Demux/5 -> Terminator_12/1
  Demux/6 -> Mux/1  "pos_x"
  Demux/7 -> Mux/2  "pos_y"
  Demux/8 -> Mux/3  "pos_z"
  Demux/10 -> Terminator_17/1
  Demux/11 -> Terminator_18/1
  Demux/12 -> Acceleration_[m/s2]/1
  Demux/13 -> Terminator_20/1
  Demux/14 -> Terminator_21/1
  Demux/15 -> Terminator_22/1
  Demux/16 -> Terminator_23/1
  Demux/17 -> compas converter/1(rotz [rad])
  Demux/18 -> Terminator_25/1
  Demux/19 -> Terminator_26/1
  Demux/20 -> Terminator_27/1
  Demux/21 -> Terminator_28/1
  Demux/22 -> Terminator_29/1
  Demux/23 -> Terminator_30/1
  Demux/9 -> Velocity_[m/s]/1
  Demux/24 -> warning_signal_id/1
  Demux/25 -> maneuvre_id/1
  Demux/26 -> vehicle_type/1
  Demux/27 -> brakingcapacity/1
  Demux/28 -> vehicle_size/1
  xyz2GPS/1 -> Demux1/1
  Demux1/1 -> GPS_pos_lat_[deg]/1
  Demux1/2 -> GPS_pos_long_[deg]/1
  Demux1/3 -> GPS_pos_alt_[m]/1
  Mux/1 -> xyz2GPS/1
  AntennaR/1 -> Reorder/1(In)
  Reorder/1(Out) -> Demux/1
  Demux/29 -> Bus Creator/1  "spare_1"
  Demux/30 -> Bus Creator/2  "spare_2"
  Demux/31 -> Bus Creator/3  "spare_3"
  Demux/32 -> Bus Creator/4  "spare_4"
  Demux/33 -> Bus Creator/5  "spare_5"
  Demux/34 -> Bus Creator/6  "spare_6"
  Demux/35 -> Bus Creator/7  "spare_7"
  Demux/36 -> Bus Creator/8  "spare_8"
  Demux/37 -> Bus Creator/9  "spare_9"
  Demux/38 -> Bus Creator/10  "spare_10"
  Demux/39 -> Bus Creator/11  "spare_11"
  Demux/40 -> Bus Creator/12  "spare_12"
  Demux/41 -> Bus Creator/13  "spare_13"
  Demux/42 -> Bus Creator/14  "spare_14"
  Demux/43 -> Bus Creator/15  "spare_15"
  Demux/44 -> Bus Creator/16  "spare_16"
  Demux/45 -> Bus Creator/17  "spare_17"
  Demux/46 -> Bus Creator/18  "spare_18"
  Demux/47 -> Bus Creator/19  "spare_19"
  Demux/48 -> Bus Creator/20  "spare_20"
  Demux/49 -> Bus Creator/21  "spare_21"
  Demux/50 -> Bus Creator/22  "spare_22"
  Demux/51 -> Bus Creator/23  "spare_23"
  Demux/52 -> Bus Creator/24  "spare_24"
  Demux/53 -> Bus Creator/25  "spare_25"
  Demux/54 -> Bus Creator/26  "spare_26"
  Demux/55 -> Bus Creator/27  "spare_27"
  Demux/56 -> Bus Creator/28  "spare_28"
  Demux/57 -> Bus Creator/29  "spare_29"
  Demux/58 -> Bus Creator/30  "spare_30"
  Demux/59 -> Bus Creator/31  "spare_31"
  Demux/60 -> Bus Creator/32  "spare_32"
  Demux/61 -> Bus Creator/33  "spare_33"
  Demux/62 -> Bus Creator/34  "spare_34"
  Demux/63 -> Bus Creator/35  "spare_35"
  Demux/64 -> Bus Creator/36  "spare_36"
  Demux/65 -> Bus Creator/37  "spare_37"
  Demux/66 -> Bus Creator/38  "spare_38"
  Demux/67 -> Bus Creator/39  "spare_39"
  Demux/91 -> Bus Creator/63  "spare_63"
  Demux/90 -> Bus Creator/62  "spare_62"
  Demux/89 -> Bus Creator/61  "spare_61"
  Demux/88 -> Bus Creator/60  "spare_60"
  Demux/87 -> Bus Creator/59  "spare_59"
  Demux/68 -> Bus Creator/40  "spare_40"
  Demux/69 -> Bus Creator/41  "spare_41"
  Demux/70 -> Bus Creator/42  "spare_42"
  Demux/71 -> Bus Creator/43  "spare_43"
  Demux/72 -> Bus Creator/44  "spare_44"
  Demux/73 -> Bus Creator/45  "spare_45"
  Demux/74 -> Bus Creator/46  "spare_46"
  Demux/75 -> Bus Creator/47  "spare_47"
  Demux/76 -> Bus Creator/48  "spare_48"
  Demux/77 -> Bus Creator/49  "spare_49"
  Demux/78 -> Bus Creator/50  "spare_50"
  Demux/79 -> Bus Creator/51  "spare_51"
  Demux/80 -> Bus Creator/52  "spare_52"
  Demux/81 -> Bus Creator/53  "spare_53"
  Demux/82 -> Bus Creator/54  "spare_54"
  Demux/83 -> Bus Creator/55  "spare_55"
  Demux/84 -> Bus Creator/56  "spare_56"
  Demux/85 -> Bus Creator/57  "spare_57"
  Demux/86 -> Bus Creator/58  "spare_58"

== system Demo_DSRC_BSM_I_and_II_Message_cs/Ford_Fiesta_1/SELF_Demux/compas converter ==
  rotz [rad] : Inport
  cart2compas : Subsystem
  rad2deg : Gain  Gain=180/pi
  heading [deg] : Outport
  wires:
  cart2compas/1(heading [deg]) -> heading [deg]/1
  rotz [rad]/1 -> rad2deg/1
  rad2deg/1 -> cart2compas/1(Angle [deg])

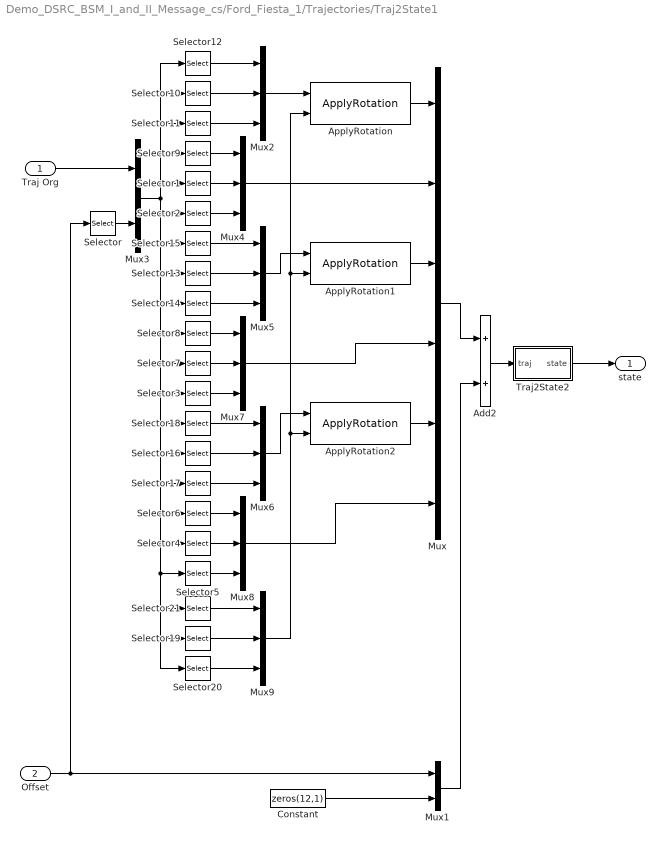
== system Demo_DSRC_BSM_I_and_II_Message_cs/Ford_Fiesta_1/Trajectories/Traj2State1 ==
  Traj Org : Inport
  Offset : Inport  Port=2
  Add2 : Sum
  ApplyRotation : PreScanSimulinkLibrary/ApplyRotation  SystemSampleTime=-1
  ApplyRotation1 : PreScanSimulinkLibrary/ApplyRotation  SystemSampleTime=-1
  ApplyRotation2 : PreScanSimulinkLibrary/ApplyRotation  SystemSampleTime=-1
  Constant : Constant  Value=zeros(12,1)
  Mux : Mux  Inputs=6
  Mux1 : Mux  Inputs=2
  Mux{2,4..9} (7 alike) : Mux  Inputs=3
  Mux3 : Mux  Inputs=2
  Selector : Selector  InputPortWidth=6  IndexOptions=Index vector (dialog)  Indices=[4 5 6]  OutputSizes=1
  Selector1 : Selector  InputPortWidth=21  IndexOptions=Index vector (dialog)  Indices=[5]  OutputSizes=1
  Selector10 : Selector  InputPortWidth=21  IndexOptions=Index vector (dialog)  Indices=[2]  OutputSizes=1
  Selector11 : Selector  InputPortWidth=21  IndexOptions=Index vector (dialog)  Indices=[3]  OutputSizes=1
  Selector12 : Selector  InputPortWidth=21  IndexOptions=Index vector (dialog)  Indices=[1]  OutputSizes=1
  Selector13 : Selector  InputPortWidth=21  IndexOptions=Index vector (dialog)  Indices=[8]  OutputSizes=1
  Selector14 : Selector  InputPortWidth=21  IndexOptions=Index vector (dialog)  Indices=[9]  OutputSizes=1
  Selector15 : Selector  InputPortWidth=21  IndexOptions=Index vector (dialog)  Indices=[7]  OutputSizes=1
  Selector16 : Selector  InputPortWidth=21  IndexOptions=Index vector (dialog)  Indices=[14]  OutputSizes=1
  Selector17 : Selector  InputPortWidth=21  IndexOptions=Index vector (dialog)  Indices=[15]  OutputSizes=1
  Selector18 : Selector  InputPortWidth=21  IndexOptions=Index vector (dialog)  Indices=[13]  OutputSizes=1
  Selector19 : Selector  InputPortWidth=21  IndexOptions=Index vector (dialog)  Indices=[20]  OutputSizes=1
  Selector2 : Selector  InputPortWidth=21  IndexOptions=Index vector (dialog)  Indices=[6]  OutputSizes=1
  Selector20 : Selector  InputPortWidth=21  IndexOptions=Index vector (dialog)  Indices=[21]  OutputSizes=1
  Selector21 : Selector  InputPortWidth=21  IndexOptions=Index vector (dialog)  Indices=[19]  OutputSizes=1
  Selector3 : Selector  InputPortWidth=21  IndexOptions=Index vector (dialog)  Indices=[12]  OutputSizes=1
  Selector4 : Selector  InputPortWidth=21  IndexOptions=Index vector (dialog)  Indices=[17]  OutputSizes=1
  Selector5 : Selector  InputPortWidth=21  IndexOptions=Index vector (dialog)  Indices=[18]  OutputSizes=1
  Selector6 : Selector  InputPortWidth=21  IndexOptions=Index vector (dialog)  Indices=[16]  OutputSizes=1
  Selector7 : Selector  InputPortWidth=21  IndexOptions=Index vector (dialog)  Indices=[11]  OutputSizes=1
  Selector8 : Selector  InputPortWidth=21  IndexOptions=Index vector (dialog)  Indices=[10]  OutputSizes=1
  Selector9 : Selector  InputPortWidth=21  IndexOptions=Index vector (dialog)  Indices=[4]  OutputSizes=1
  Traj2State2 : Subsystem
  state : Outport
  wires:
  Mux9/1 -> ApplyRotation2/2, ApplyRotation1/2, ApplyRotation/2
  Selector20/1 -> Mux9/3
  Selector19/1 -> Mux9/2
  Selector21/1 -> Mux9/1
  Selector5/1 -> Mux8/3
  Selector4/1 -> Mux8/2
  Selector6/1 -> Mux8/1
  Mux8/1 -> Mux/6
  Mux6/1 -> ApplyRotation2/1
  Mux7/1 -> Mux/4
  ApplyRotation2/1 -> Mux/5
  Selector3/1 -> Mux7/3
  Selector7/1 -> Mux7/2
  Selector8/1 -> Mux7/1
  Mux4/1 -> Mux/2
  Mux5/1 -> ApplyRotation1/1
  ApplyRotation1/1 -> Mux/3
  Mux2/1 -> ApplyRotation/1
  ApplyRotation/1 -> Mux/1
  Selector2/1 -> Mux4/3
  Selector1/1 -> Mux4/2
  Selector9/1 -> Mux4/1
  Selector17/1 -> Mux6/3
  Selector16/1 -> Mux6/2
  Selector18/1 -> Mux6/1
  Selector14/1 -> Mux5/3
  Selector13/1 -> Mux5/2
  Selector15/1 -> Mux5/1
  Selector11/1 -> Mux2/3
  Selector10/1 -> Mux2/2
  Selector12/1 -> Mux2/1
  Mux3/1 -> Selector8/1, Selector7/1, Selector3/1, Selector18/1, Selector16/1, Selector17/1, Selector6/1, Selector20/1, Selector19/1, Selector21/1, Selector5/1, Selector4/1, Selector14/1, Selector13/1, Selector15/1, Selector2/1, Selector1/1, Selector9/1, Selector12/1, Selector10/1, Selector11/1
  Mux1/1 -> Add2/2
  Constant/1 -> Mux1/2
  Add2/1 -> Traj2State2/1(traj)
  Selector/1 -> Mux3/2
  Traj Org/1 -> Mux3/1
  Offset/1 -> Mux1/1, Selector/1
  Mux/1 -> Add2/1
  Traj2State2/1(state) -> state/1

== system Demo_DSRC_BSM_I_and_II_Message_cs/Ford_Fiesta_1/Trajectories/Trajectory_2 ==
  From Workspace : FromWorkspace  VariableName=trajectory  SampleTime=TimeStep  OutputAfterFinalValue=Holding final value
  From Workspace1 : FromWorkspace  VariableName=trajectory  SampleTime=TimeStep  OutputAfterFinalValue=Setting to zero
  Mux : Mux  Inputs=2
  Selector1 : Selector  InputPortWidth=24  IndexOptions=Index vector (dialog)  Indices=[7:18]  OutputSizes=1
  Selector9 : Selector  InputPortWidth=24  IndexOptions=Index vector (dialog)  Indices=[1:6]  OutputSizes=1
  trajectory : Outport
  wires:
  Selector1/1 -> Mux/2
  Selector9/1 -> Mux/1
  Mux/1 -> trajectory/1
  From Workspace1/1 -> Selector1/1
  From Workspace/1 -> Selector9/1

== system Demo_DSRC_BSM_I_and_II_Message_cs/Mazda_RX8_1/Basic Safety Message II/BSM-II Creator ==
  ThrottlePositon : Inport
  ExteriorLights : Inport  Port=2
  CrumbData : Inport  Port=3
  itemCnt : Inport  Port=4
  Confidence : Inport  Port=5
  RadiusOfCurve : Inport  Port=6
  EventFlag : Inport  Port=7
  Bus Creator : BusCreator  Inputs='ThrottlePosition','ExteriorLights'  OutDataTypeStr=Bus: VehicleStatus
  Bus Creator1 : BusCreator  Inputs='CrumbData','itemCnt'  OutDataTypeStr=Bus: PathHistory
  Bus Creator2 : BusCreator  Inputs='Confidence','RadiusOfCurve'  OutDataTypeStr=Bus: PathPrediction
  Bus Creator3 : BusCreator  Inputs='PathPrediction','PathHistory','EventFlag'  OutDataTypeStr=Bus: VehicleSafetyExtension
  Bus Creator4 : BusCreator  Inputs='VehicleStatus','VehicleSafetyExtension'  OutDataTypeStr=Bus: BSMII
  BSMII : Outport
  wires:
  Bus Creator/1 -> Bus Creator4/1  "VehicleStatus"
  ThrottlePositon/1 -> Bus Creator/1  "ThrottlePosition"
  ExteriorLights/1 -> Bus Creator/2  "ExteriorLights"
  CrumbData/1 -> Bus Creator1/1  "CrumbData"
  itemCnt/1 -> Bus Creator1/2  "itemCnt"
  Bus Creator1/1 -> Bus Creator3/2  "PathHistory"
  Confidence/1 -> Bus Creator2/1  "Confidence"
  RadiusOfCurve/1 -> Bus Creator2/2  "RadiusOfCurve"
  Bus Creator2/1 -> Bus Creator3/1  "PathPrediction"
  EventFlag/1 -> Bus Creator3/3  "EventFlag"
  Bus Creator3/1 -> Bus Creator4/2  "VehicleSafetyExtension"
  Bus Creator4/1 -> BSMII/1

== system Demo_DSRC_BSM_I_and_II_Message_cs/Mazda_RX8_1/Basic Safety Message II/BSM-II Unpacker ==
  BSMII : Inport
  Bus Selector : BusSelector  OutputSignals=VehicleStatus.ThrottlePosition,VehicleStatus.ExteriorLights,VehicleSafetyExtension.PathPrediction.Confidence,VehicleSafetyExtension.PathPrediction.RadiusOfCurve,VehicleSafetyExtension.PathHistory.CrumbData,VehicleSafetyExtension.PathHistory.itemCnt,VehicleSafetyExtension.EventFlag
  Embedded MATLAB Function : Stateflow chart  TreatAsAtomicUnit=on
  Eventflag : Outport
  itemCnt : Outport  Port=2
  RadiusOfCurve : Outport  Port=3
  Confidence : Outport  Port=4
  ExteriorLights : Outport  Port=5
  ThrottlePosition : Outport  Port=6
  CrumbData_DoubleVector : Outport  Port=7
  wires:
  BSMII/1 -> Bus Selector/1  "BSMII"
  Bus Selector/5 -> Embedded MATLAB Function/1(u)  "<CrumbData>"
  Bus Selector/7 -> Eventflag/1  "<EventFlag>"
  Bus Selector/6 -> itemCnt/1  "<itemCnt>"
  Bus Selector/4 -> RadiusOfCurve/1  "<RadiusOfCurve>"
  Bus Selector/3 -> Confidence/1  "<Confidence>"
  Bus Selector/2 -> ExteriorLights/1  "<ExteriorLights>"
  Bus Selector/1 -> ThrottlePosition/1  "<ThrottlePosition>"
  Embedded MATLAB Function/1(y) -> CrumbData_DoubleVector/1

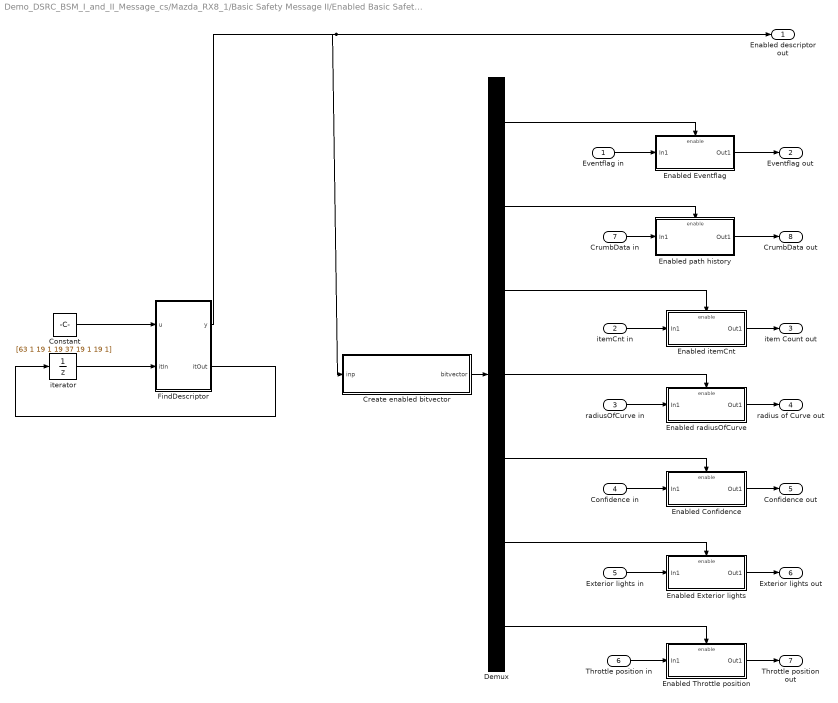
== system Demo_DSRC_BSM_I_and_II_Message_cs/Mazda_RX8_1/Basic Safety Message II/Enabled Basic Safety Message I and II ==
  Eventflag in : Inport
  itemCnt in : Inport  Port=2
  radiusOfCurve in : Inport  Port=3
  Confidence in : Inport  Port=4
  Exterior lights in : Inport  Port=5
  Throttle position in : Inport  Port=6
  CrumbData in : Inport  Port=7
  Constant : Constant  Value=[63 1 19 1 19 37 19 1 19 1]
      settings: PreSaveFcn=|
      | val=evalin('base','DSRCT_vectenabled_Str');
      | h=gcb;
      | set_param(h,'value',val);
  Create enabled bitvector : Stateflow chart  TreatAsAtomicUnit=on
  Demux : Demux  Outputs=7
  Enabled Confidence : Subsystem  TreatAsAtomicUnit=on
  Enabled Eventflag : Subsystem  TreatAsAtomicUnit=on
  Enabled Exterior lights : Subsystem  TreatAsAtomicUnit=on
  Enabled itemCnt : Subsystem  TreatAsAtomicUnit=on
  Enabled radiusOfCurve : Subsystem  TreatAsAtomicUnit=on
  Enabled Throttle position : Subsystem  TreatAsAtomicUnit=on
  Enabled path history : Subsystem  TreatAsAtomicUnit=on
  FindDescriptor : Stateflow chart  TreatAsAtomicUnit=on
  iterator : UnitDelay  X0=1  SampleTime=-1
  Enabled descriptor out : Outport
  Eventflag out : Outport  Port=2
  item Count out : Outport  Port=3
  radius of Curve out : Outport  Port=4
  Confidence out : Outport  Port=5
  Exterior lights out : Outport  Port=6
  Throttle position out : Outport  Port=7
  CrumbData out : Outport  Port=8
  wires:
  FindDescriptor/2(itOut) -> iterator/1
  iterator/1 -> FindDescriptor/2(itIn)
  FindDescriptor/1(y) -> Enabled descriptor out/1, Create enabled bitvector/1(inp)
  Enabled path history/1(Out1) -> CrumbData out/1
  CrumbData in/1 -> Enabled path history/1(In1)
  Create enabled bitvector/1(bitvector) -> Demux/1
  Enabled Eventflag/1(Out1) -> Eventflag out/1
  Enabled radiusOfCurve/1(Out1) -> radius of Curve out/1
  Eventflag in/1 -> Enabled Eventflag/1(In1)
  itemCnt in/1 -> Enabled itemCnt/1(In1)
  radiusOfCurve in/1 -> Enabled radiusOfCurve/1(In1)
  Confidence in/1 -> Enabled Confidence/1(In1)
  Exterior lights in/1 -> Enabled Exterior lights/1(In1)
  Throttle position in/1 -> Enabled Throttle position/1(In1)
  Demux/2 -> Enabled path history/Enable
  Constant/1 -> FindDescriptor/1(u)
  Demux/1 -> Enabled Eventflag/Enable
  Demux/3 -> Enabled itemCnt/Enable
  Demux/4 -> Enabled radiusOfCurve/Enable
  Demux/5 -> Enabled Confidence/Enable
  Enabled Confidence/1(Out1) -> Confidence out/1
  Demux/6 -> Enabled Exterior lights/Enable
  Enabled Exterior lights/1(Out1) -> Exterior lights out/1
  Demux/7 -> Enabled Throttle position/Enable
  Enabled Throttle position/1(Out1) -> Throttle position out/1
  Enabled itemCnt/1(Out1) -> item Count out/1

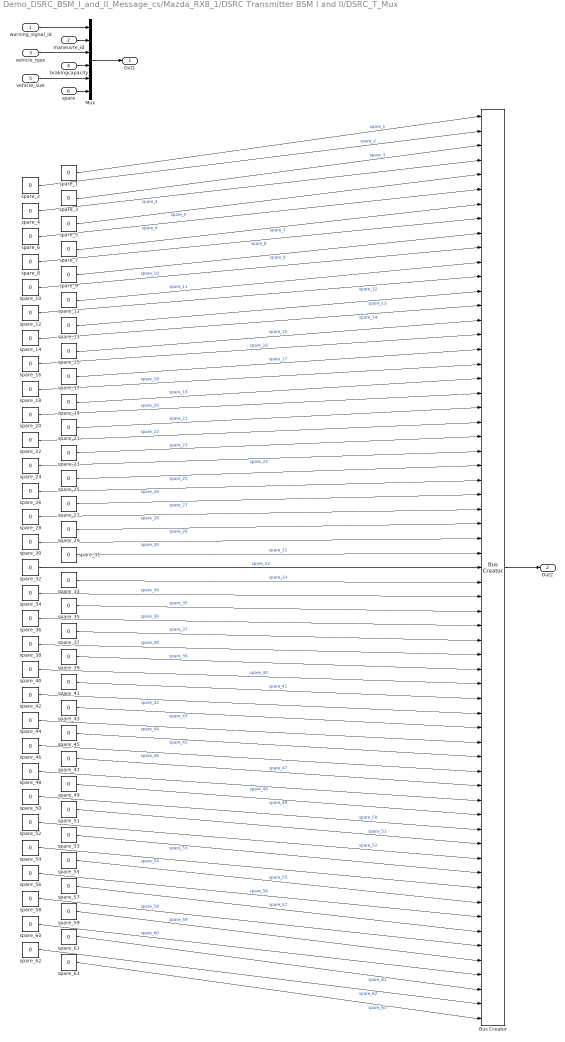
== system Demo_DSRC_BSM_I_and_II_Message_cs/Mazda_RX8_1/DSRC Transmitter BSM I and II/DSRC_T_Mux ==
  warning_signal_id : Inport
  maneuvre_id : Inport  Port=2
  vehicle_type : Inport  Port=3
  brakingcapacity : Inport  Port=4
  vehicle_size : Inport  Port=5
  spare : Inport  Port=6
  Bus Creator : BusCreator  Inputs=63
  Mux : Mux  Inputs=6
  spare_{1..63} (63 alike) : Constant  Value=0
  Out1 : Outport
  Out2 : Outport  Port=2
  wires:
  warning_signal_id/1 -> Mux/1
  maneuvre_id/1 -> Mux/2
  vehicle_type/1 -> Mux/3
  brakingcapacity/1 -> Mux/4
  vehicle_size/1 -> Mux/5
  Mux/1 -> Out1/1
  spare/1 -> Mux/6
  spare_19/1 -> Bus Creator/19  "spare_19"
  spare_18/1 -> Bus Creator/18  "spare_18"
  spare_17/1 -> Bus Creator/17  "spare_17"
  spare_16/1 -> Bus Creator/16  "spare_16"
  spare_15/1 -> Bus Creator/15  "spare_15"
  spare_14/1 -> Bus Creator/14  "spare_14"
  spare_13/1 -> Bus Creator/13  "spare_13"
  spare_12/1 -> Bus Creator/12  "spare_12"
  spare_11/1 -> Bus Creator/11  "spare_11"
  spare_10/1 -> Bus Creator/10  "spare_10"
  spare_9/1 -> Bus Creator/9  "spare_9"
  spare_8/1 -> Bus Creator/8  "spare_8"
  spare_7/1 -> Bus Creator/7  "spare_7"
  spare_6/1 -> Bus Creator/6  "spare_6"
  spare_5/1 -> Bus Creator/5  "spare_5"
  spare_4/1 -> Bus Creator/4  "spare_4"
  spare_1/1 -> Bus Creator/1  "spare_1"
  spare_2/1 -> Bus Creator/2  "spare_2"
  spare_3/1 -> Bus Creator/3  "spare_3"
  spare_20/1 -> Bus Creator/20  "spare_20"
  spare_21/1 -> Bus Creator/21  "spare_21"
  spare_22/1 -> Bus Creator/22  "spare_22"
  spare_23/1 -> Bus Creator/23  "spare_23"
  spare_24/1 -> Bus Creator/24  "spare_24"
  spare_25/1 -> Bus Creator/25  "spare_25"
  spare_26/1 -> Bus Creator/26  "spare_26"
  spare_27/1 -> Bus Creator/27  "spare_27"
  spare_28/1 -> Bus Creator/28  "spare_28"
  spare_29/1 -> Bus Creator/29  "spare_29"
  spare_30/1 -> Bus Creator/30  "spare_30"
  spare_31/1 -> Bus Creator/31  "spare_31"
  spare_32/1 -> Bus Creator/32  "spare_32"
  spare_33/1 -> Bus Creator/33  "spare_33"
  spare_34/1 -> Bus Creator/34  "spare_34"
  spare_35/1 -> Bus Creator/35  "spare_35"
  spare_36/1 -> Bus Creator/36  "spare_36"
  spare_37/1 -> Bus Creator/37  "spare_37"
  spare_38/1 -> Bus Creator/38  "spare_38"
  spare_39/1 -> Bus Creator/39  "spare_39"
  spare_40/1 -> Bus Creator/40  "spare_40"
  spare_41/1 -> Bus Creator/41  "spare_41"
  spare_42/1 -> Bus Creator/42  "spare_42"
  spare_43/1 -> Bus Creator/43  "spare_43"
  spare_44/1 -> Bus Creator/44  "spare_44"
  spare_45/1 -> Bus Creator/45  "spare_45"
  spare_46/1 -> Bus Creator/46  "spare_46"
  spare_47/1 -> Bus Creator/47  "spare_47"
  spare_48/1 -> Bus Creator/48  "spare_48"
  spare_49/1 -> Bus Creator/49  "spare_49"
  spare_50/1 -> Bus Creator/50  "spare_50"
  spare_51/1 -> Bus Creator/51  "spare_51"
  spare_52/1 -> Bus Creator/52  "spare_52"
  spare_53/1 -> Bus Creator/53  "spare_53"
  spare_54/1 -> Bus Creator/54  "spare_54"
  spare_55/1 -> Bus Creator/55  "spare_55"
  spare_56/1 -> Bus Creator/56  "spare_56"
  spare_57/1 -> Bus Creator/57  "spare_57"
  spare_58/1 -> Bus Creator/58  "spare_58"
  spare_59/1 -> Bus Creator/59  "spare_59"
  spare_60/1 -> Bus Creator/60  "spare_60"
  spare_61/1 -> Bus Creator/61  "spare_61"
  spare_62/1 -> Bus Creator/62  "spare_62"
  spare_63/1 -> Bus Creator/63  "spare_63"
  Bus Creator/1 -> Out2/1

== system Demo_DSRC_BSM_I_and_II_Message_cs/Mazda_RX8_1/Radius and confidence computation/Center point of the bend ==
  note: q^2
  note: Determines coordinates [x,y] of the center
      | of the bend on which car drives
  R : Inport
  delta_Phi : Inport  Port=2
  "[x1,y1]" : Inport  Port=3
  "[x2,y2]" : Inport  Port=4
  Add : Sum  Inputs=-+
  Dot Product1 : DotProduct  InputSameDT=on  OutDataTypeStr=Inherit: Inherit via internal rule
  If Action Subsystem : Subsystem  TreatAsAtomicUnit=on
  If Action Subsystem1 : Subsystem  TreatAsAtomicUnit=on
  If1 : If  NumInputs=2  IfExpression=(u1 ~= 0) & (u2 ~= 0)
  Merge : Merge
  Center point : Outport
  wires:
  "[x1,y1]"/1 -> Add/1, If Action Subsystem/5("[x1,y1]")
  Add/1 -> Dot Product1/1, Dot Product1/2, If Action Subsystem/4(diff_[x,y])
  "[x2,y2]"/1 -> Add/2, If Action Subsystem/6("[x2,y2]")
  Dot Product1/1 -> If1/1, If Action Subsystem/3(q^2)
  If1/1 -> If Action Subsystem/Action
  If1/2 -> If Action Subsystem1/Action
  R/1 -> If1/2, If Action Subsystem/1(R)
  delta_Phi/1 -> If Action Subsystem/2(delta_Phi)
  If Action Subsystem/1("[xp,yp]") -> Merge/1
  If Action Subsystem1/1("[xp,yp]") -> Merge/2
  Merge/1 -> Center point/1

== system Demo_DSRC_BSM_I_and_II_Message_cs/Mazda_RX8_1/Radius and confidence computation/Confidence level ==
  note: Value of confidance computed
      |    with use of yaw rate derivative
  Yaw rate [deg/s] : Inport
  Abs : Abs
  Derivative approximation : Subsystem
  FIR filter1 : Subsystem
  FIR filter2 : Subsystem
  Lookup Table confidence level1 : Lookup  InputValues=[ 0, 0.5, 1, 1.5, 2, 2.5, 5, 10, 15, 20 ]  Table=[ 100, 90, 80, 70, 60, 50, 40, 30, 20, 0 ]  LookUpMeth=Interpolation-Use End Values
  Rate Transition : RateTransition  Integrity=off  OutPortSampleTime=GPS_sample_time
  Confidence [%] : Outport
  wires:
  Derivative approximation/1(d(YawRate)) -> FIR filter1/1(In1)
  Lookup Table confidence level1/1 -> FIR filter2/1(In1)
  FIR filter1/1(Out1) -> Abs/1
  Yaw rate [deg/s]/1 -> Rate Transition/1
  Rate Transition/1 -> Derivative approximation/1(yaw rate)
  FIR filter2/1(Out1) -> Confidence [%]/1
  Abs/1 -> Lookup Table confidence level1/1

== system Demo_DSRC_BSM_I_and_II_Message_cs/Mazda_RX8_1/Radius and confidence computation/Degrees2Radians ==
  Iat1d : Inport
  Iong1d : Inport  Port=2
  heading1d : Inport  Port=3
  lat2d : Inport  Port=4
  long2d : Inport  Port=5
  heading2d : Inport  Port=6
  Degrees to Radians : simulink_extras/Transformations/Degrees to Radians  SystemSampleTime=-1
  Demux : Demux  Outputs=6
  Mux : Mux  Inputs=6
  lat1r : Outport
  long1r : Outport  Port=2
  heading1r : Outport  Port=3
  lat2r : Outport  Port=4
  long2r : Outport  Port=5
  heading2r : Outport  Port=6
  wires:
  Iat1d/1 -> Mux/1
  Iong1d/1 -> Mux/2
  lat2d/1 -> Mux/4
  long2d/1 -> Mux/5
  Mux/1 -> Degrees to Radians/1
  Degrees to Radians/1 -> Demux/1
  Demux/1 -> lat1r/1
  Demux/2 -> long1r/1
  Demux/4 -> lat2r/1
  Demux/5 -> long2r/1
  Demux/6 -> heading2r/1
  Demux/3 -> heading1r/1
  heading2d/1 -> Mux/6
  heading1d/1 -> Mux/3

== system Demo_DSRC_BSM_I_and_II_Message_cs/Mazda_RX8_1/Radius and confidence computation/Heading angle conversion ==
  note: Transcrips value of heading
      |    angle to interval from 0 to <360 degrees
  H_in [deg] : Inport
  Constant : Constant  Value=360  SampleTime=GPS_sample_time
  Math Function : Math  Operator=mod  SaturateOnIntegerOverflow=on
  H_out [deg] : Outport
  wires:
  Constant/1 -> Math Function/2
  H_in [deg]/1 -> Math Function/1
  Math Function/1 -> H_out [deg]/1
